simulink model "pure_design_vol1"  (R2024b)
settings: Solver=VariableStepAuto  StartTime=0.0  StopTime=10  RelTol=1e-3
libraries: spsDiodeLib x7, spsSeriesRLCBranchLib x3, spsPWMGeneratorDCDCLib x1, spsDCMachineLib x1, spsDCVoltageSourceLib x1, spsIGBTDiodeLib x1, spsCurrentMeasurementLib x1, spsThreePhaseSourceLib x1, sps_lib x1
settings Model: Creator=pipil  LastModifiedBy=pipil

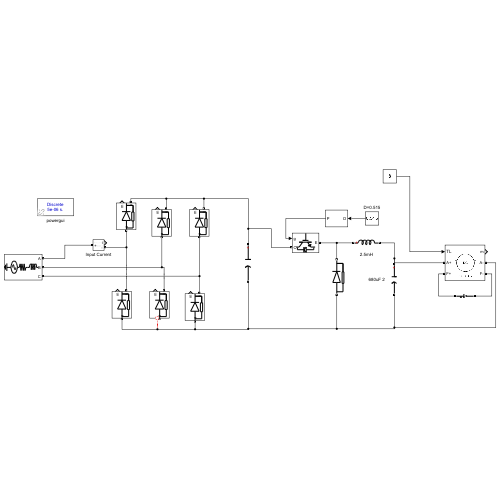
[thumbnail: Simulink's stored preview of the top-level diagram]
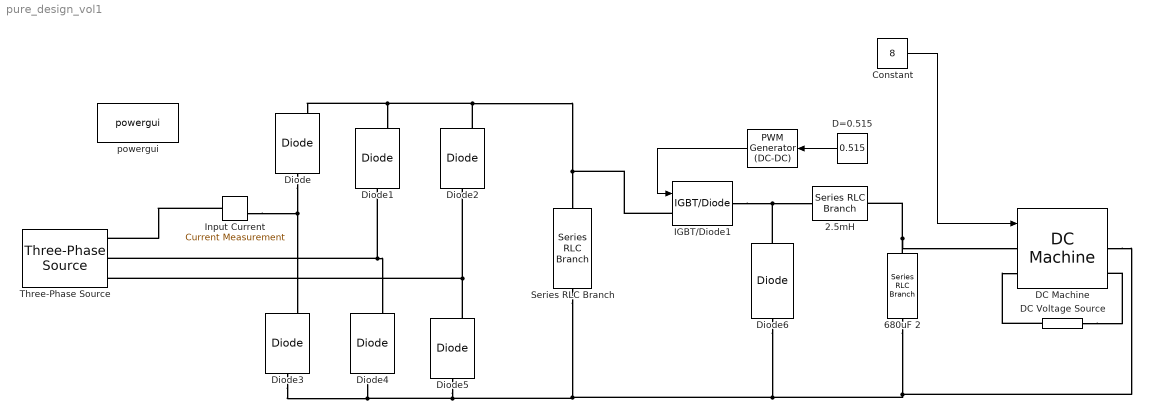
== system pure_design_vol1 ==
  "  " : spsPWMGeneratorDCDCLib/PWM Generator (DC-DC)  Fsw=500  Ts=0
  2.5mH : spsSeriesRLCBranchLib/Series RLC Branch  LConnTagsString=__new0  RConnTagsString=__new0  BranchType=L  Resistance=1  Inductance=2.5e-3  SetiL0=off  InitialCurrent=0  Capacitance=1e-6  Setx0=off  InitialVoltage=0  Measurements=None
  680uF 2 : spsSeriesRLCBranchLib/Series RLC Branch  LConnTagsString=__new0  RConnTagsString=__new0  BranchType=C  Resistance=1  Inductance=1e-3  SetiL0=off  InitialCurrent=0  Capacitance=680e-6  Setx0=off  InitialVoltage=0  Measurements=None
  Constant : Constant  Value=8
  D=0.515 : Constant  Value=0.515
  DC Machine : spsDCMachineLib/DC Machine  PresetModel=No  MechanicalLoad=Torque TL  FieldType=Wound  ShowDetailedParameters=on  MeasurementBus=on  RLa="[ 0.8  0.0125]"  RLf="[ 210  23]"  Laf=1.8  MachineConstant=Torque constant (N.m/A)  Ke=1.8  Kt=1.8  J=0.1  Bm=0  Tf=0.2  w0=1  Ifinit=1.04761904756944  TsPowergui=0  TsBlock=-1
  DC Voltage Source : spsDCVoltageSourceLib/DC Voltage Source  Amplitude=220  Measurements=None
  Diode{,1..5} (6 alike) : spsDiodeLib/Diode  Ron=1e-10  Lon=0  Vf=0  IC=0  UseSnubber=0  Rs=500  Cs=1e-10  Measurements=on
  Diode6 : spsDiodeLib/Diode  Ron=0.001  Lon=0  Vf=0.8  IC=0  UseSnubber=0  Rs=500  Cs=250e-9  Measurements=off
  IGBT/Diode1 : spsIGBTDiodeLib/IGBT//Diode  Ron=1e-3  Rs=1e5  Cs=inf  Measurements=off
  Input Current : spsCurrentMeasurementLib/Current Measurement  PhasorSimulation=off  OutputType=Complex  PSBequivalent=0
  Series RLC Branch : spsSeriesRLCBranchLib/Series RLC Branch  LConnTagsString=__new0  RConnTagsString=__new0  BranchType=C  Resistance=1  Inductance=47e-3  SetiL0=off  InitialCurrent=0  Capacitance=47e-6  Setx0=off  InitialVoltage=0  Measurements=None
  Three-Phase Source : spsThreePhaseSourceLib/Three-Phase Source  InternalConnection=Yg  VoltagePhases=off  Voltage=220*sqrt(3)  PhaseAngle=0  Voltage_phases=[25e3 25e3 25e3]/sqrt(3)  PhaseAngles_phases=[0 -120 +120]  Frequency=50  NonIdealSource=on  SpecifyImpedance=off  Resistance=0.8929  Inductance=16.58e-3  ShortCircuitLevel=100e6  BaseVoltage=25e3  XRratio=7  BusType=swing  Pref=10e3  Qref=0  Prefabc=[10e3, 10e3, 10e3]  Qrefabc=[0, 0, 0]  Qmin=-inf  Qmax=inf
  powergui : sps_lib/powergui  Priority=1  SimulationMode=Discrete  SampleTime=5e-6  frequency=60  Iterations=50  frequencyindice=0  Pbase=100e6  ErrMax=1e-4  UnitsV=kV  UnitsW=MW  buscounter=0  FunctionMessages=off  echomessages=off  EnableUseOfTLC=off  CurrentSourceSwitches=off  DisableSnubberDevices=off  DisableRonSwitches=off  DisableVfSwitches=off  DisplayEquations=off  AutomaticDiscreteSolvers=off  SolverType=Tustin/Backward Euler (TBE)  Interpol=off  ExternalGateDelay=off  methode=off  Ts=100  x0status=blocks  SPID=on  SwTol=0  HookPort=off  NonlinearTolerance=1e-4  nMaxIteration=100  ContinueOnMaxIteration=off  RestoreLinks=warning  ResistiveCurrentMeasurement=off  Frange=[0:2:500]  Ylog=off  Xlog=on  ShowGrid=off  save=off  variable=ZData  structure=0  ZoomFFT=off  StartTime=0.0  cycles=1  DisplayStyle=1  fundamental=60  FreqAxis=off  MaxFrequency=1000  frequencyindicesteady=1  RmsSteady=1  display=off
  wires:
  Constant/1 -> DC Machine/1
  D=0.515/1 -> "  "/1
  "  "/1 -> IGBT/Diode1/1
  connections:
  Diode2/RConn1 -- IGBT/Diode1/LConn1 -- Series RLC Branch/LConn1 -- Diode/RConn1 -- Diode1/RConn1
  680uF 2/RConn1 -- DC Machine/RConn1 -- Diode6/LConn1 -- Diode5/LConn1 -- Diode3/LConn1 -- Series RLC Branch/RConn1
  Diode/LConn1 -- Diode3/RConn1 -- Input Current/RConn1
  Three-Phase Source/RConn2 -- Diode4/RConn1 -- Diode1/LConn1
  Three-Phase Source/RConn3 -- Diode2/LConn1 -- Diode5/RConn1
  Input Current/LConn1 -- Three-Phase Source/RConn1
  Diode6/RConn1 -- IGBT/Diode1/RConn1 -- 2.5mH/LConn1
  2.5mH/RConn1 -- DC Machine/LConn1 -- 680uF 2/LConn1
  DC Voltage Source/RConn1 -- DC Machine/LConn2
  DC Voltage Source/LConn1 -- DC Machine/RConn2
